simulink library "Ampere_Library"  (R2022b)
settings: Solver=FixedStepDiscrete  StartTime=0  StopTime=10.0  RelTol=1e-3  EnableMultiTasking=on
undefined symbols (not defined in the file or in its folder): A_INST_double, Dem_EventStatusType, ECU_AMBIENT_TEMPERATURE, SET_ECU_AMBIENT_TEMPERATURE, SlDemoSign, Std_ReturnType
libraries: simulink x13
(part 3 of 10)

== system Ampere_Library/User_Defined_Libraries/Discrete ==
  note: Specific
  note: Freezing
  note: Ramping
  note: Integrators
  note: Filters
  note: Delays
  note: Discrete
  A_1stO_Der_Fltr_Cont : Subsystem  Tag=[LIB]  mask(A_1stO_Der_Fltr_Cont){dOut_by_dt=on, SaturateOnOverflow=off, tolerance=double tol - eps('double'), user_tol=0}
      mask prompts: dOut_by_dt "Tick if dOut_by_dt output is required"; SaturateOnOverflow "Saturate on integer overflow"; tolerance "Tolerance for DivisionByZero"; user_tol "User Defined Tolerance"
      mask help:
      | This block performs the first order filter operation and the derivation on it.
      |
      | At the start of simulation, Input 'Init_val', will be the value of output 'Out'.
      | From the next sample time the filter operation will start based on the values of Inputs 'In' and 'Tau'.
      | The derivative calculation is done on the filtered signal which will be produced by the output 'dOut_by_dt'.
      |
      | Continuity:
      | - If 'Continuity' Input is true
      | When the Input 'Reset' is true, After the initial time step, output 'dOut_by_dt' will be set same as the Input 'IC_Derivative' value and Output 'Out' will be calculated as per the below formula
      |
      | Out = In - Tau*IC_Derivative.
      |
      | - If 'Continuity' Input is false
      | When the Input 'Reset' is true, the Output 'Out' will be set as per input 'Init_val' value and the derivative Output 'dOut_by_dt' is set to 0.
      |
      | When "Tick if dOut_by_dt output is required" parameter is Selected, then both output ports 'Out' and  'dOut_by_dt' will be available. Else only output port 'Out' will be available.
      |
      | For Integers,
      | Overflow is handled by enabling "Tick if Saturation is required".
      |
      | For Double/Single,
      | User must ensure to give values within maximum and minimum value of (single/double)datatype.Otherwise it will results in overflow.
      mask init:
      | %% Init values
      | ConstZero = 0;
      | UDEIC_zero = 0;
      | 
      | %% Update the block dOut_by_dt as outport or terminator depending of the mask value
      | if strcmp(get_param(gcb,'dOut_by_dt'),'off')
      |     already_exist = find_system(gcb,'LookUnderMasks','all','FollowLinks','on','SearchDepth',1,'BlockType','Terminator','Name','dOut_by_dt');
      |     if isempty(already_exist)
      |         h = replace_block(gcb,'Followlinks','on','name','dOut_by_dt','built-in/terminator','noprompt');
      |         set_param(h{1},'ShowName','off');
      |     end
      | else
      |     already_exist = find_system(gcb,'LookUnderMasks','all','FollowLinks','on','SearchDepth',1,'BlockType','Outport','Name','dOut_by_dt');
      |     if isempty(already_exist)
      |         h = replace_block(gcb,'Followlinks','on','name','dOut_by_dt','built-in/Outport','noprompt');
      |         set_param(h{1},'backgroundcolor','orange');
      |         set_param(h{1},'ShowName','on');
      |     end
      | end
      | 
      | %% Compute the tolerance
      | switch tolerance
      |     case 1
      |         tol = eps('double');
      |     case 2
      |         tol = eps('single');
      |     case 3
      |         tol = 0;
      |     case 4
      |         tol = user_tol;
      | end
      | 
      | %% Create the infos to display below the block depending of the Mask Options
      | % Always display MaskType
      | Attrib = '%<MaskType>';
      | % Conditionnally adding Tolerance value
      | if strcmp(get_param(gcb,'tolerance'),'User Defined tol')
      |     Attrib = [Attrib '\nTolerance = %<user_tol>'];
      | end
      | % Conditionnally adding Saturation
      | if strcmp(get_param(gcb,'SaturateOnOverflow'),'on')
      |     Attrib = [Attrib '\nSAT = on'];
      | end
      | % Update the display
      | set_param(gcb,'AttributesFormatString',Attrib);
      settings: AttributesFormatString=%<MaskType>
      mask TypeOptions SaturateOnOverflow: MinMax1/SaturateOnIntegerOverflow | Switch1/SaturateOnIntegerOverflow | Switch2/SaturateOnIntegerOverflow | Switch3/SaturateOnIntegerOverflow | Switch4/SaturateOnIntegerOverflow | Product/SaturateOnIntegerOverflow | Product1/SaturateOnIntegerOverflow | Sum/SaturateOnIntegerOverflow | Sum1/SaturateOnIntegerOverflow | Sum2/SaturateOnIntegerOverflow | Sum3/SaturateOnIntegerOverflow | A_UnitDelayExternalIC/Init/SaturateOnIntegerOverflow | A_DivisionByZero/Switch/SaturateOnIntegerOverflow | A_DivisionByZero/Divide/SaturateOnIntegerOverflow | A_DivisionByZero/Abs1/SaturateOnIntegerOverflow
      mask TypeOptions tolerance: double tol - eps('double') | single tol - eps('single') | Absolute Zero tol | User Defined tol
      mask Callback tolerance:
      | %% Make visible or not the Tolerance Value (update 4th element of MaskVisibilities)
      | MaskVisibilities = get_param(gcb,'MaskVisibilities');
      | if strcmp(get_param(gcb,'tolerance'),'User Defined tol')
      |     MaskVisibilities{4} = 'on';
      | else
      |     MaskVisibilities{4} = 'off';
      | end
      | set_param(gcb,'MaskVisibilities',MaskVisibilities);
      mask Display: disp('Discrete FirstOrder\nFilter Resettable\nDerivative Continuity');
  A_1stOrder_Derivative_Filter : Subsystem  Tag=[LIB]  mask(A_1stOrder_Derivative_Filter){dOut_by_dt=on, SaturateOnOverflow=off, tolerance=double tol - eps('double'), user_tol=0}
      mask prompts: dOut_by_dt "Tick if dOut_by_dt output is required"; SaturateOnOverflow "Saturate on integer overflow"; tolerance "Tolerance for DivisionByZero"; user_tol "User Defined Tolerance"
      mask help:
      | The block performs the first order filter operation and the derivation on it.
      | For the start of simulation input 'Init_val', will be the output 'Out' value, and from the next sample time the filter operation will happen, depending on the values of the inputs 'In' and 'Tau'.
      | The derivative calculation is done on the filtered signal and given by the output 'dOut_by_dt'.
      | If the input 'Reset' is true the output is forced to 'Init_val' and the derivative to 0.
      mask init:
      | %% Internal parameters
      | ConstZero = 0;
      | UDEIC_zero = 0;
      | 
      | %% Update the block dOut_by_dt as outport or terminator depending of the mask value
      | if strcmp(get_param(gcb,'dOut_by_dt'),'off')
      |     already_exist = find_system(gcb,'LookUnderMasks','all','FollowLinks','on','SearchDepth',1,'BlockType','Terminator','Name','dOut_by_dt');
      |     if isempty(already_exist)
      |         h = replace_block(gcb,'Followlinks','on','name','dOut_by_dt','built-in/terminator','noprompt');
      |         set_param(h{1},'ShowName','off');
      |     end
      | else
      |     already_exist = find_system(gcb,'LookUnderMasks','all','FollowLinks','on','SearchDepth',1,'BlockType','Outport','Name','dOut_by_dt');
      |     if isempty(already_exist)
      |         h = replace_block(gcb,'Followlinks','on','name','dOut_by_dt','built-in/Outport','noprompt');
      |         set_param(h{1},'backgroundcolor','orange');
      |         set_param(h{1},'ShowName','on');
      |     end
      | end
      | 
      | %% Compute the tolerance
      | switch tolerance
      |     case 1
      |         tol = eps('double');
      |     case 2
      |         tol = eps('single');
      |     case 3
      |         tol = 0;
      |     case 4
      |         tol = user_tol;
      | end
      | 
      | %% Create the infos to display below the block depending of the Mask Options
      | % Always display MaskType
      | Attrib = '%<MaskType>';
      | % Conditionnally adding Tolerance value
      | if strcmp(get_param(gcb,'tolerance'),'User Defined tol')
      |     Attrib = [Attrib '\nTolerance = %<user_tol>'];
      | end
      | % Conditionnally adding Saturation
      | if strcmp(get_param(gcb,'SaturateOnOverflow'),'on')
      |     Attrib = [Attrib '\nSAT = on'];
      | end
      | % Update the display
      | set_param(gcb,'AttributesFormatString',Attrib);
      settings: AttributesFormatString=%<MaskType>
      mask TypeOptions SaturateOnOverflow: MinMax1/SaturateOnIntegerOverflow | Product/SaturateOnIntegerOverflow | Sum/SaturateOnIntegerOverflow | Sum1/SaturateOnIntegerOverflow | Sum2/SaturateOnIntegerOverflow | Switch2/SaturateOnIntegerOverflow | Switch3/SaturateOnIntegerOverflow | A_UnitDelayExternalIC/Init/SaturateOnIntegerOverflow | A_DivisionByZero/Abs1/SaturateOnIntegerOverflow | A_DivisionByZero/Divide/SaturateOnIntegerOverflow | A_DivisionByZero/Switch/SaturateOnIntegerOverflow
      mask TypeOptions tolerance: double tol - eps('double') | single tol - eps('single') | Absolute Zero tol | User Defined tol
      mask Callback tolerance:
      | %% Make visible or not the Tolerance Value (update 4th element of MaskVisibilities)
      | MaskVisibilities = get_param(gcb,'MaskVisibilities');
      | if strcmp(get_param(gcb,'tolerance'),'User Defined tol')
      |     MaskVisibilities{4} = 'on';
      | else
      |     MaskVisibilities{4} = 'off';
      | end
      | set_param(gcb,'MaskVisibilities',MaskVisibilities);
      mask Display:
      | %% Display info on the icon
      | fprintf('Discrete FirstOrder\nFilter Resettable');
  A_DiagnosticFilter : Subsystem  Tag=[LIB]  mask(A_DiagnosticFilter){WaitTime=3, in_NA=5, DefaultValue=-10, DiagnosticValue=1, TsDiag=0.1, UpperLimit=realmax('double'), LowerLimit=0, tolerance=double tol - eps('double'), user_tol=0}
      mask prompts: WaitTime "Waiting time (s)"; in_NA "Unavailable value"; DefaultValue "Default value (when block is disabled)"; DiagnosticValue "Diagnostic value (when input is declared unavailable)"; TsDiag "Sample Time used for calculation, should not be inherited (-1)."; UpperLimit "SAT max for Saturation Block"; LowerLimit "SAT min for Saturation Block"; tolerance "Tolerance for Unavailable Value"; user_tol "User Defined Tolerance"
      mask help:
      | When the input value 'in' is the unavailable value, this block freezes its output 'out' during the waiting time specified.
      | It returns the diagnostic value afterwards. If the input is unavailable at initialization, this block returns directly the diagnostic value.
      | When the block is disabled, it returns a default value.
      mask init:
      | %% Internal parameters
      | IniVal = 0;
      | Cons1 = 1;
      | Cons2 = 2;
      | Cons3 = 3;
      | Normal_mode = Cons1;
      | TsDiag_init = -TsDiag;
      | 
      | %% Compute tolerance
      | switch tolerance
      |     case 1
      |         tol = eps('double');
      |     case 2
      |         tol = eps('single');
      |     case 3
      |         tol = 0;
      |     case 4
      |         tol = user_tol;
      | end
      settings: AttributesFormatString=%<MaskType>
      mask TypeOptions tolerance: double tol - eps('double') | single tol - eps('single') | Absolute Zero tol | User Defined tol
      mask Callback tolerance:
      | %% Make visible or not the Tolerance Value (update 9th element of MaskVisibilities)
      | MaskVisibilities = get_param(gcb,'MaskVisibilities');
      | if strcmp(get_param(gcb,'tolerance'),'User Defined tol')
      |     MaskVisibilities{9} = 'on';
      | else
      |     MaskVisibilities{9} = 'off';
      | end
      | set_param(gcb,'MaskVisibilities',MaskVisibilities);
      mask Display:
      | %% Display info on the icon
      | fprintf('(8 params in the mask)')
  A_DiscreteInt_Ext_SAT : Subsystem  Tag=[LIB]  mask(A_DiscreteInt_Ext_SAT){SaturateOnOverflow=off}
      mask prompts: SaturateOnOverflow "Saturate on integer overflow"
      mask help:
      | Discrete integrator, based on Euler's method :
      |  y[k] = y[k-1] + Ts.u[k-1]
      |
      |  Where,
      |  Ts = sample time
      | The Input 'Ts' is used for the the value of Ts in the calculations.
      |
      | Reset is based on the rising of the external signal.
      |
      | The calculated Output 'out' is bound with :
      |   - The Input 'sat_max' for upper limit
      |   - The Input 'sat_min' for lower limit
      mask init:
      | %% Internal parameters
      | IniVal = 0;
      | Input_IC = 0;
      settings: AttributesFormatString=%<MaskType>
      mask TypeOptions SaturateOnOverflow: MinMax/SaturateOnIntegerOverflow | MinMax1/SaturateOnIntegerOverflow | Product/SaturateOnIntegerOverflow | Sum1/SaturateOnIntegerOverflow | Switch/SaturateOnIntegerOverflow
      mask Callback SaturateOnOverflow:
      | %% Display SaturateOnOverflow only when set to on
      | Attrib = '%%<MaskType>';
      | if strcmp(get(gcbh,'SaturateOnOverflow'),'on')
      |     Attrib = [Attrib '\nSAT = on'];
      | end
      | set(gcbh,'AttributesFormatString',sprintf(Attrib));
      mask Display:
      | %% Display info on the icon
      | fprintf('Discrete Integrator\nExternal Saturation');
  A_DiscreteIntegrator : Subsystem  Tag=[LIB]  mask(A_DiscreteIntegrator){K=0.23, Ts=0.1, reset=level, sat_max=100, sat_min=0, SaturateOnOverflow=off}
      mask prompts: K "gain"; Ts "Sample Time used for calculation, should not be inherited (-1)."; reset "external reset"; sat_max "upper saturation limit"; sat_min "lower saturation limit"; SaturateOnOverflow "Saturate on integer overflow"
      mask help:
      | The DiscreteIntegrator block uses the Euler's method for the integration.
      |
      | y[k] = y[k-1] + K *Ts *u[k-1]
      |
      | Where,
      | y=out
      | u=in
      | K = gain
      | Ts = sample time
      | k= Time step
      |
      | If external reset is not used, provide 'reset' input with 0
      mask init:
      | %% Internal Parameter
      | IniVal = 0;
      | 
      | %% Based on reset value GotoTag updated
      | if reset==1
      |     set_param([gcb '/VarFrom'],'GotoTag','ext_reset_and');
      | else
      |     set_param([gcb '/VarFrom'],'GotoTag','ext_reset_or');
      | end
      | %% Getting the value of upper and lower sat limit
      | stmax = get_param(gcbh, 'sat_max');
      | stmin = get_param(gcbh, 'sat_min');
      | 
      | %% Convert char arrays to objects
      | if all(isstrprop(stmax,"digit")|isstrprop(stmax,"punct"))
      |     % stmax: For handling numeric values
      |     stmax = str2double(stmax);
      | else
      |     % stmax: For handling MWS,base workspace and sldd
      |     mdlWks = get_param(bdroot(gcbh), 'ModelWorkspace');
      |     if hasVariable(mdlWks, stmax)
      |         stmax = getVariable(mdlWks, stmax);
      |     else
      |         stmax = Simulink.data.evalinGlobal(bdroot(gcbh), stmax);
      |     end
      | end
      | if all(isstrprop(stmin,"digit")|isstrprop(stmin,"punct"))
      |     % stmin: For handling numeric values
      |     stmin = str2double(stmin);
      | else
      |     % stmin: For handling MWS,base workspace and sldd
      |     mdlWks = get_param(bdroot(gcbh), 'ModelWorkspace');
      |     if hasVariable(mdlWks, stmin)
      |         stmin = getVariable(mdlWks, stmin);
      |     else
      |         stmin = Simulink.data.evalinGlobal(bdroot(gcbh), stmin);
      |     end
      | end
      | 
      | %% Convert Simulink Parameter objects to values
      | if ~isempty(regexp(class(stmax),'Parameter', 'once'))
      |     stmax = stmax.Value;
      | end
      | if ~isempty(regexp(class(stmin),'Parameter', 'once'))
      |     stmin = stmin.Value;
      | end
      | 
      | %% Do not allow non-numeric values, non-scalars or not-finite values
      | assert(isnumeric(stmax) && isscalar(stmax) && isfinite(stmax), 'Numeric finite scalar expected for stmax');
      | assert(isnumeric(stmin) && isscalar(stmin) && isfinite(stmin), 'Numeric finite scalar expected for stmin');
      | 
      | %% Do not allow max < min
      | assert(stmax >= stmin, 'Ensure upper limit is greater than lower limit');
      settings: AttributesFormatString=|
      | %<MaskType>
      | external reset = %<reset>
      mask TypeOptions reset: rising | level
      mask TypeOptions SaturateOnOverflow: MinMax/SaturateOnIntegerOverflow | MinMax1/SaturateOnIntegerOverflow | Product/SaturateOnIntegerOverflow | Product1/SaturateOnIntegerOverflow | Sum1/SaturateOnIntegerOverflow | Switch/SaturateOnIntegerOverflow
      mask Callback SaturateOnOverflow:
      | if strcmp(get_param(gcb,'SaturateOnOverflow'),'on')
      |     % Display the SaturateOnOverflow parameter
      |     set_param(gcb, 'AttributesFormatString', sprintf('%%<MaskType>\nexternal reset = %%<reset>\nSAT = on'));
      | else
      |     % Do not display the SaturateOnOverflow parameter
      |     set_param(gcb, 'AttributesFormatString', sprintf('%%<MaskType>\nexternal reset = %%<reset>'));
      | end
      mask Display:
      | %% Display info on the icon
      | fprintf('y[k]=y[k-1]+K*Ts*u[k-1]\nK = %s\nTs = %s\nUp lim : %s\nLow lim : %s',...
      |     get_param(gcb,'K'),...
      |     get_param(gcb,'Ts'),...
      |     get_param(gcb,'sat_max'),...
      |     get_param(gcb,'sat_min'));
  A_DownFreezing : Subsystem  Tag=[LIB]  mask(A_DownFreezing){init=0.1, SaturateOnOverflow=off}
      mask prompts: init "Initial condition"; SaturateOnOverflow "Saturate on integer overflow"
      mask help:
      | The block compares the previous and present value of the input 'in' and outputs minimum of the two values in output 'out'.
      | The initial value for input is specified by 'Initial Condition' parameter in mask.
      settings: AttributesFormatString=%<MaskType>
      mask TypeOptions SaturateOnOverflow: MinMax/SaturateOnIntegerOverflow
      mask Callback SaturateOnOverflow:
      | if strcmp(get_param(gcb,'SaturateOnOverflow'),'on')
      |     % Display the SaturateOnOverflow parameter
      |     set_param(gcb, 'AttributesFormatString', sprintf('%%<MaskType>\nSAT = on'));
      | else
      |     % Do not display the SaturateOnOverflow parameter
      |     set_param(gcb, 'AttributesFormatString', sprintf('%%<MaskType>'));
      | end
      mask Display:
      | %% Display info on the icon
      | fprintf('IC = %s', get_param(gcb,'init'));
  A_FILTER1ST : Subsystem  Tag=[LIB]  mask(A_FILTER1ST){initial_value=0, OutputDataT=double}
      mask prompts: OutputDataT "Internal Product Operation DataType"
      mask help:
      | First order filter
      |
      | output = (input - output_old)* filter_parameter + output_old
      |
      | Initial_value
      |   output_old initial value
      |
      | Inputs:
      |     input : input signal
      |     filter_parameter : parameter of the filter with 0 <= filter_parameter <= 1
      |     initial
      |             1 : Initialize (output = input)
      |             0 : The filter operates using the previous formulation
      |
      | Outputs:
      |     output : output of the filter
      |
      | Note :
      | The input 'initial' shall be a boolean
      | This block will support only Double datatype.
      mask init:
      | %% Internal parameters
      | Low = 0;
      | Up = 1;
      | output_satmin = -1.79769e+308; % least minimum double value on the negative side
      | output_satmax = 1.79769e+308; % Real positive double value on the positive side
      | 
      | %% Set output data type of internal Product block
      | set_param([gcb '/Product'], 'OutDataTypeStr', get_param(gcbh,'OutputDataT'));
      settings: AttributesFormatString=|
      | %<MaskType>
      | Init = %<initial_value>
  A_FirstOrderClim : Subsystem  Tag=[LIB]  mask(A_FirstOrderClim){resolution=eps, enable_port=on, default_value=1.5, contrl_value=1e-15, prod_OutDataTypeStr=Inherit: Inherit via internal rule, tolerance_value=double tol - eps('double'), userdef_tol=0.1}
      mask prompts: resolution "Signal resolution"; enable_port "Make it as Enable Subsystem"; default_value "Default value (when disabled)"; contrl_value "Control Value if Den <= Tolerance"; prod_OutDataTypeStr "Simulink:blkprm_prompts:OUTPUT_UNIFIEDDATATYPE"; tolerance_value "Tolerance"; userdef_tol "User Defined Tolerance"
      mask help:
      | The FirstOrderClim block performs the first order filter operation as explained below.
      | 1. When Make it as Enable Subsystem is selected & When 'Enable' is 1:
      |     a.Initial Output value will be 'Init' converted at the specific resolution.
      |     b.Further Output will be calculated based on Output formula mentioned below.
      | 2. When Make it as Enable Subsystem is selected & When 'Enable' is 0:
      |      a. Output will always be the 'Default Value' given in the mask parameter.
      | 3. When Make it as Enable Subsystem is de-selected:
      |      a.Initial Output value will be 'Init' converted at the specific resolution
      |      b.Further Output will be calculated based on Output formula mentioned below.
      | 4.Output formula
      |     a.Out_tmp(k) =    [(In * T_by_Tau ) + Out_tmp(k-1)]/(T_by_Tau + 1)
      |     b.Out(k) = [Round (Out_tmp(k) / Signal resolution)]* Signal resolution
      mask init:
      | %% Internal Parameters
      | IniVal = 0;
      | RF0 = 0;
      | RF5 = 0.5;
      | RF1 = 1;
      | 
      | %% Updating the content with or without the Enable block
      | if strcmp(get_param(gcb,'enable_port'),'on')
      |     % Check if there is no Enable block
      |     if isempty(find_system(gcb,'Searchdepth',1,'FollowLinks','on','LookUnderMasks','all','Name','enableport1'))
      |         % Add the enable block
      |         add_block('built-in/EnablePort',[gcb '/enableport1'],...
      |             'MakeNameUnique','on',...
      |             'StatesWhenEnabling','reset',...
      |             'position','[380 65 400 85]',...
      |             'ShowName','on',...
      |             'AttributesFormatString',sprintf('%%<StatesWhenEnabling>'));
      |         % Update the properties of the Outport
      |         set_param([gcb '/Out'],'AttributesFormatString',sprintf('%%<OutputWhenDisabled>\nInit = %%<InitialOutput>'),...
      |             'outputWhenDisabled','reset',...
      |             'InitialOutput','default_value');
      |     end
      | else % Without Enable block
      |     if ~isempty(find_system(gcb,'Searchdepth',1,'FollowLinks','on','LookUnderMasks','all','Name','enableport1'))
      |         % Delete the Enable block
      |         delete_block(get_param([gcb '/enableport1'],'handle'));
      |         % Update the properties of the Outport
      |         set_param([gcb '/Out'],'AttributesFormatString','',...
      |             'outputWhenDisabled','held',...
      |             'InitialOutput','[]');
      |     end
      | end
      | 
      | %% Compute the tolerance
      | switch tolerance_value
      |     case 1
      |         tol = eps('double');
      |     case 2
      |         tol = eps('single');
      |     case 3
      |         tol = 0;
      |     case 4
      |         tol = userdef_tol;
      | end
      | 
      | %% Create the infos to display below the block depending of the Mask Options
      | % Always display MaskType
      | Attrib = '%<MaskType>';
      | % Conditionnally adding Default value
      | if strcmp(get_param(gcb,'enable_port'),'on')
      |     Attrib = [Attrib '\nDef val = %<default_value>'];
      | end
      | % Always display Control value
      | Attrib = [Attrib '\nCtrl val = %<contrl_value>'];
      | % Conditionnally adding Tolerance
      | if strcmp(get_param(gcb,'tolerance_value'),'User Defined tol')
      |     Attrib = [Attrib '\nTol = %<userdef_tol>'];
      | end
      | % Update the display
      | set_param(gcb,'AttributesFormatString',Attrib);
      settings: AttributesFormatString=%<MaskType>\nDef val = %<default_value>\nCtrl val = %<contrl_value>
      mask Callback enable_port:
      | %% Make visible or not the Default Value (update 3rd element of MaskVisibilities)
      | MaskVisibilities = get_param(gcb,'MaskVisibilities');
      | if strcmp(get_param(gcb,'enable_port'),'on')
      |     MaskVisibilities{3} = 'on';
      | else
      |     MaskVisibilities{3} = 'off';
      | end
      | set_param(gcb,'MaskVisibilities',MaskVisibilities);
      mask TypeOptions prod_OutDataTypeStr: Product1/OutDataTypeStr
      mask TypeOptions tolerance_value: double tol - eps('double') | single tol - eps('single') | Absolute Zero tol | User Defined tol
      mask Callback tolerance_value:
      | %% Make visible or not the User Defined Tolerance (update 7th element of MaskVisibilities)
      | MaskVisibilities = get_param(gcb,'MaskVisibilities');
      | if strcmp(get_param(gcb,'tolerance_value'),'User Defined tol')
      |     MaskVisibilities{7} = 'on';
      | else
      |     MaskVisibilities{7} = 'off';
      | end
      | set_param(gcb,'MaskVisibilities',MaskVisibilities);
      mask DialogControl prod_OutDataTypeStr Prompt: Output data type:
      mask Display:
      | %% Display info on the icon
      | fprintf('1st order\nfilter\nResolution = %s',get_param(gcbh,'resolution'));
  A_InvalidValue : Subsystem  Tag=[LIB]  mask(A_InvalidValue){InvalidValue=0}
      mask prompts: InvalidValue "Invalid Value"
      mask help: A_InvalidValue will output the value which is assigned in "Invalid Value" mask parameter
      settings: AttributesFormatString=%<MaskType>
      mask Display:
      | %% Display info on the icon
      | fprintf('Invalid Val:\n%s',get(gcbh,'InvalidValue'))
  A_Ramping : Subsystem  Tag=[LIB]  mask(A_Ramping){resolution=0.001, TSample=0.1, prod_OutDataTypeStr=Inherit: Inherit via back propagation}
      mask prompts: resolution "Output Signal Resolution"; TSample "Sample Time used for calculation, should not be inherited (-1)"; prod_OutDataTypeStr "Simulink:blkprm_prompts:OUTPUT_UNIFIEDDATATYPE"
      mask help:
      | The block performs the ramp up and ramp down operation, when the input "Inp" changes from low value to high value and high to low value respectively.
      | The output "Out" ramp-up  in steps of the input "SlopeInc_T" and ramp-down in steps of input "SlopeDec_T". Input "Init" is the initial value of the output "Out".
      |
      | Note: Output data type of the block has to be chosen by the user through "Output data type" mask parameter.
      mask init:
      | %% Internal parameters
      | RF0 = 0;
      | RF5 = 0.5;
      | RF1 = 1;
      | same_dt_num_of_inputs = 2;
      | UDEIC_zero = 0;
      settings: AttributesFormatString=|
      | %<MaskType>
      | Signal resolution = %<resolution>
      | Sample Time = %<TSample>
      mask Callback resolution:
      | %% Callback function to check that <resolution> parameter is greater than zero.
      | % Otherwise, a division by zero could occur
      | if str2num(get_param(gcbh, 'resolution'))<=0
      |     errordlg([{'The <Resolution> parameter''s value must be greater than 0.'} ...
      |         {'Error located in: ' gcb}], 'Resolution value error');
      | end
      mask TypeOptions prod_OutDataTypeStr: Product4/OutDataTypeStr
      mask DialogControl prod_OutDataTypeStr Prompt: Output data type:
      mask Display:
      | %% Display info on the icon
      | fprintf('Ramping');
  A_Ramping_with_EnRst : Subsystem  Tag=[LIB]  mask(A_Ramping_with_EnRst){SaturateOnOverflow=off}
      mask prompts: SaturateOnOverflow "Saturate on integer overflow"
      mask help:
      | The block performs the ramp up and ramp down operation, when the input "inp" changes from low value to high value and high to low value respectively.
      |
      | The output "out" ramp-up  in steps of the input "SlopeInc_T" and ramp-down in steps of  input "SlopeDec_T".
      |
      | Input "Init" is the initial value of the output "out".
      | The input "SlopeEna" have to be true to enable the ramp.
      | The output "out" is forced to the value of "Init" as far as the input "Reset" is true.
      |
      | Note:
      | For single/double datatype,User must ensure to give values within maximum and minimum value of (single/double)datatype.Otherwise it will result in overflow.
      |
      | For integers, Overflow is handled by enabling "Saturate on integer overflow" option.
      |
      | SlopeInc_T and SlopeDec_T values must be a positive value (Slope Magnitude). If not, then block will not behave as expected.
      mask init:
      | %% Init internal parameters
      | RF0 = 0;
      | RF5 = 0.5;
      | RF1 = 1;
      | UDEIC_zero = 0;
      settings: AttributesFormatString=%<MaskType>
      mask TypeOptions SaturateOnOverflow: Add1/SaturateOnIntegerOverflow | Add2/SaturateOnIntegerOverflow | MinMax1/SaturateOnIntegerOverflow | MinMax2/SaturateOnIntegerOverflow | Product/SaturateOnIntegerOverflow | Product1/SaturateOnIntegerOverflow | Switch1/SaturateOnIntegerOverflow | Switch2/SaturateOnIntegerOverflow | Switch/SaturateOnIntegerOverflow
      mask Callback SaturateOnOverflow:
      | if strcmp(get_param(gcb,'SaturateOnOverflow'),'on')
      |     % Display the SaturateOnOverflow parameter
      |     set_param(gcb, 'AttributesFormatString', sprintf('%%<MaskType>\nSAT = on'));
      | else
      |     % Do not display the SaturateOnOverflow parameter
      |     set_param(gcb, 'AttributesFormatString', sprintf('%%<MaskType>'));
      | end
      mask DialogControl Container Prompt: Parameters
      mask Display:
      | %% Display info on the icon
      | disp('Ramping\nEnable&Reset');
  A_TappedDelay : Subsystem  Tag=[LIB]  mask(A_TappedDelay){NoOfDelayS=4, OrderValue=Newest, init_val=5, AppendValue=on, SaturateOnOverflow=off}
      mask prompts: NoOfDelayS "No Of Delay"; OrderValue "Order output vector starting with"; init_val "Initial condition"; AppendValue "Include current input in output vector"; SaturateOnOverflow "Saturate on integer overflow for switch block"
      mask help:
      | Delay a signal by 'N' sample periods and output all the delayed versions of the signal.
      |
      | Note:
      | 1) Since 20b AMR Rules, the native Simulink Tapped Delay block is allowed and can be used.
      | 2) In 22b, the native block still doesn't support enums. Use this library block for this use case.
      mask init:
      | %% Init values
      | IniAdd = uint32(1);
      | TapdIni = uint32(0);
      | 
      | %% Check Input value
      | if NoOfDelayS == -1
      |     NoOfDelay = 1;
      | else
      |     NoOfDelay = NoOfDelayS;
      | end
      | 
      | %% Value to stop considering init value
      | A_NoOfDelay = uint32(1:NoOfDelay);
      | 
      | %% Compute "selector values" of selector blocks
      | if NoOfDelay == 1
      |     Selector = 1:NoOfDelay;
      | else
      |     Selector = 1:NoOfDelay-1;
      | end
      | % update Mux blocks Inputs values for display
      | set_param([gcb '/Mux'],'Inputs',sprintf('[1 %d]',NoOfDelay-1));
      | set_param([gcb '/Mux1'],'Inputs',sprintf('[1 %d]',NoOfDelay));
      | 
      | %% Manage the append of values for Newest/Oldest
      | Append = (2-AppendValue):NoOfDelay+1;
      | if AppendValue
      |     Order_Selec_Req = 1:(NoOfDelay+1);
      |     Order_Selec_Inv = (NoOfDelay+1):-1:1;
      | else
      |     Order_Selec_Req = 1:NoOfDelay;
      |     Order_Selec_Inv = NoOfDelay:-1:1;
      | end
      | 
      | %% Update the From block linked to the output depending of Newest/Oldest
      | if OrderValue == 1
      |     set_param([gcb '/varOrder'],'GotoTag','newest_order');
      | else
      |     set_param([gcb '/varOrder'],'GotoTag','oldest_order');
      | end
      settings: AttributesFormatString=|
      | %<MaskType>
      | IC = %<init_val>
      mask Callback NoOfDelayS:
      | % Update Tag depending on mask option NoOfDelayS
      | if (str2double(get(gcbh,'NoOfDelayS'))<=0 && str2double(get(gcbh,'NoOfDelayS'))~=-1)
      |     errorString = ['At: ' gcb '. The number of delays must be positive or -1 for inherited.'];
      |     errordlg(errorString);
      | end
      mask TypeOptions OrderValue: Newest | Oldest
      mask TypeOptions SaturateOnOverflow: Switch4/SaturateOnIntegerOverflow
      mask Display:
      | %% Display info on the icon
      | % fprintf('%d\nDelays\nOrder = %s\nInclude Input = %s',NoOfDelayS,get_param(gcbh,'OrderValue'),get_param(gcbh,'AppendValue'));
      | fprintf('%d\nDelays\n%s\nInput = %s',NoOfDelayS,get_param(gcbh,'OrderValue'),get_param(gcbh,'AppendValue'));
  A_TimeDwnFrzSatOut : Subsystem  Tag=[LIB]  mask(A_TimeDwnFrzSatOut){WaitInitTime=0, InitialValue=4294967295, FreezedValue=65535, ST=2, SaturateOnOverflow=off}
      mask prompts: WaitInitTime "Time during  initial value is frozen"; InitialValue "Initial Value"; FreezedValue "Output Frozen Value"; ST "Sample Time (Used for calculation, should not be inherited (-1))."; SaturateOnOverflow "Saturate on integer overflow"
      mask help: Timer down saturated output provides "Initial Value" at the output, until the "Time During Initial Value is Frozen". After the timer elapses, it will give the input value as output or frozen value as output, when the input is smaller than the "Frozen Value".
      mask init:
      | %% Internal Parameter
      | IniVal = uint32(0);
      settings: AttributesFormatString=|
      | %<MaskType>
      | IC = %<InitialValue>
      mask TypeOptions SaturateOnOverflow: Add1/SaturateOnIntegerOverflow | Add2/SaturateOnIntegerOverflow | Switch/SaturateOnIntegerOverflow | Switch1/SaturateOnIntegerOverflow | Switch2/SaturateOnIntegerOverflow | Switch3/SaturateOnIntegerOverflow | Switch4/SaturateOnIntegerOverflow
      mask Callback SaturateOnOverflow:
      | if strcmp(get_param(gcb,'SaturateOnOverflow'),'on')
      |     % Display the SaturateOnOverflow parameter
      |     set_param(gcb, 'AttributesFormatString', sprintf('%%<MaskType>\nIC = %%<InitialValue>\nSAT = on'));
      | else
      |     % Do not display the SaturateOnOverflow parameter
      |     set_param(gcb, 'AttributesFormatString', sprintf('%%<MaskType>\nIC = %%<InitialValue>'));
      | end
      mask Display:
      | %% Display info on the icon
      | fprintf('Timed Down Freezing\nSaturated Output')
  A_UnitDelayExternalIC : Subsystem  Tag=[LIB]  mask(A_UnitDelayExternalIC){SaturateOnOverflow=off}
      mask prompts: SaturateOnOverflow "Saturate on integer overflow"
      mask help:
      | The block's output 'y' is the input signal 'u' delayed by one sample period.
      | Note:The initial condition is given by the input 'IC'.
      settings: AttributesFormatString=%<MaskType>
      mask TypeOptions SaturateOnOverflow: Init/SaturateOnIntegerOverflow
      mask Callback SaturateOnOverflow:
      | %% Create the info to display below the block
      | Attrib = '%<MaskType>';
      | % Conditionnally display the SaturateOnOverflow parameter
      | if strcmp(get_param(gcb,'SaturateOnOverflow'),'on')
      |     Attrib = [Attrib '\nSAT = on'];
      | end
      | set_param(gcb, 'AttributesFormatString', Attrib);
      mask Display:
      | %% Plot the symbol 1/z on the icon
      | dpoly(1,[1 0],'z')
  A_UnitDelayResettable : Subsystem  Tag=[LIB]  mask(A_UnitDelayResettable){SaturateOnOverflow=off}
      mask prompts: SaturateOnOverflow "Saturate on integer overflow"
      mask help:
      | The output of this block is the input signal "u" delayed by one sample period.
      | The initial condition is given by the signal IC.
      | When Reset signal is True, initial condition given by the signal "IC" is the output.
      mask init:
      | %% Internal parameter
      | UDEIC_zero = 0;
      settings: AttributesFormatString=%<MaskType>
      mask TypeOptions SaturateOnOverflow: Switch/SaturateOnIntegerOverflow
      mask Callback SaturateOnOverflow:
      | %% Create the info to display below the block
      | Attrib = '%<MaskType>';
      | % Conditionnally display the SaturateOnOverflow parameter
      | if strcmp(get_param(gcb,'SaturateOnOverflow'),'on')
      |     Attrib = [Attrib '\nSAT = on'];
      | end
      | set_param(gcb, 'AttributesFormatString', Attrib);
      mask Display:
      | %% Plot the symbol 1/z on the icon
      | dpoly(1,[1 0],'z')

== system Ampere_Library/User_Defined_Libraries/FlipFlop ==
  note: Obsolete
  note: Flip-Flop for all use cases
  note: Flip-Flop
  A_SRFlipFlop_Mask_Cust : Subsystem  Tag=[LIB]  mask(A_SRFlipFlop_Mask_Cust){Init=true, Indeterminate_Condition_out=true}
      mask prompts: Init "Initial Condition"; Indeterminate_Condition_out "Output when S=TRUE and R=TRUE"
      mask help:
      | The S-R flip-flop also known as a set-reset flip-flop.
      | The truth table for this block is:
      |
      |  Set  ReSet    |   Out
      |  --------------------
      |  0      0          |   Init Value or Prev Output
      |  0      1          |   0
      |  1      0          |   1
      |  1      1          |   UserDefined
      |
      | When both inputs Set (S) and ReSet (R) are true, the output is set to 'Output when S=TRUE and R=TRUE'.
      | This allows the user to specify the FlipFlop as Set priority (output true) or Reset priority (output false).
      | The initial value for the output is given by the mask parameter 'Initial Condition'.
      mask init:
      | %% Update Init Value
      | switch Init
      |     case 1
      |         IC = true;
      |     case 2
      |         IC = false;
      | end
      | 
      | %% Update tags and values of blocks for the intermediate condition
      | switch Indeterminate_Condition_out
      |     case 1
      |         % Set prioritary
      |         set_param([gcb '/ConstantCb1'],'Value','true');
      |         set_param([gcb '/ConstantCb2'],'Value','false');
      |         set_param([gcb '/FromCb1'],'GotoTag','Set');
      |         set_param([gcb '/FromCb2'],'GotoTag','ReSet');
      |     case 2
      |         % Reset prioritary
      |         set_param([gcb '/ConstantCb1'],'Value','false');
      |         set_param([gcb '/ConstantCb2'],'Value','true');
      |         set_param([gcb '/FromCb1'],'GotoTag','ReSet');
      |         set_param([gcb '/FromCb2'],'GotoTag','Set');
      | end
      settings: AttributesFormatString=%<MaskType>
      mask TypeOptions Init: true | false
      mask TypeOptions Indeterminate_Condition_out: true | false
      mask Display:
      | %% Display info on the icon
      | fprintf('Indeterm = %s\nIC = %s',...
      |     upper(char(extract(get_param(gcbh,'Indeterminate_Condition_out'),1))),...
      |     upper(char(extract(get_param(gcbh,'Init'),1))));
  A_SRFlipFlop_indeter_F : Subsystem  Tag=[LIB]  mask(A_SRFlipFlop_indeter_F){}
      mask help:
      | **************************************************************
      | OBSOLETE
      | Use instead A_SRFlipFlop_Mask_Cust configured as:
      |    Initial Condition set to false
      |    Output when S=TRUE and R=TRUE set to false
      | **************************************************************
      |
      | When the input ("set") gets the value 1 (TRUE), the output ("flag") will be set to 1 (TRUE)
      |
      | When the input ("clear") gets the value 0 (FALSE), the output ("flag") will be set to 0 (FALSE)
      |
      | When both inputs get the value 1 (TRUE), the output ("flag") will be set to 0 (FALSE)
      |
      | When both input get the value 0 (FALSE), the output ("flag") will maintain its previous value.
      mask init:
      | %% Internal parameter
      | init_flag_set = 0;
      settings: AttributesFormatString=%<MaskType>
